simulink model "MPC_Lateral_Control_Model"  (R2021a)
settings: Solver=VariableStepAuto  StartTime=0.0  StopTime=Ts  RelTol=1e-3
InitFcn:
  | MPC_init
StopFcn:
  | simulation_plots_week6
values from neighbouring files (symbols this model uses):
  Vx = 25    [LCA_init.m]    (also in MPC_init.m = 10; week6_init.m = 30)
libraries: mpclib x1
settings Model: Creator=User  LastModifiedBy=User

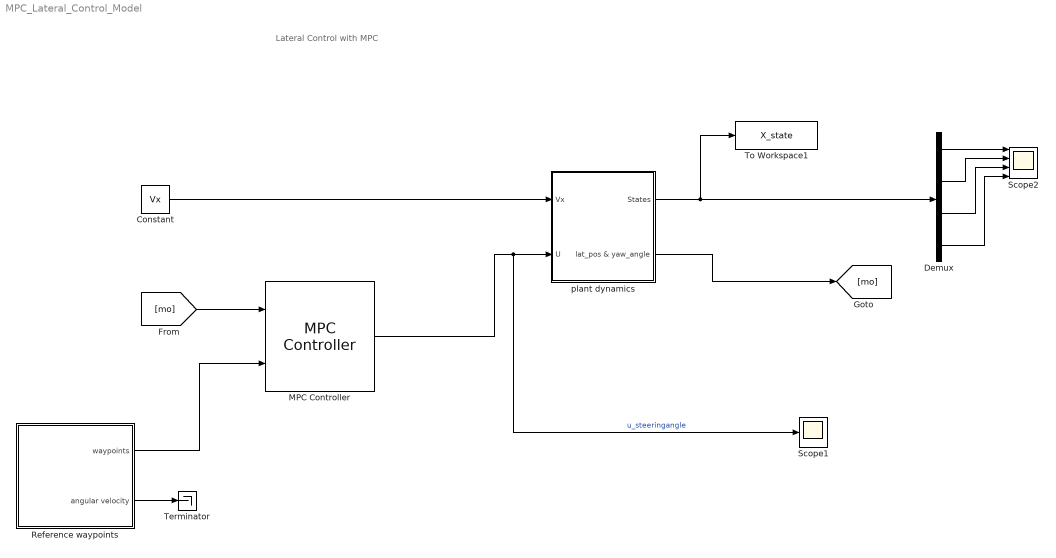
== system MPC_Lateral_Control_Model ==
  note: Lateral Control with MPC
  Constant : Constant  Value=Vx
  Demux : Demux
  MPC Controller : mpclib/MPC Controller  SCDEnableBlockLinearizationSpecification=on  mpcobj=mpc1  is_multiple=0  enable_value=0  return_u0=off  updateMPCinCallerWorkspace=on  md_inport=off  mv_inport=off  uref_inport=off  return_cost=off  return_mvseq=off  return_qpstatus=off  return_xseq=off  return_state=off  return_ovseq=off  state_inport=off  umin_inport=off  umax_inport=off  ymin_inport=off  ymax_inport=off  cc_inport=off  ywt_inport=off  uwt_inport=off  duwt_inport=off  rhoeps_inport=off  pm_inport=off  MaximumP=10  HorizonChoice=FixedHorizon  n_ts=0.1  n_p=10  n_mv=1  n_md=0  n_ud=0  n_mo=2  n_uo=0  BlockDataType=double  SampleTimeInherited=off  switch_inport=off
  Reference waypoints : Subsystem
  Scope1 : Scope
  Scope2 : Scope  NumInputPorts=4
  Terminator : Terminator
  To Workspace1 : ToWorkspace  VariableName=X_state  SampleTime=-1
  plant dynamics : Subsystem
  wires:
  Reference waypoints/1(waypoints) -> MPC Controller/2
  plant dynamics/2(lat_pos & yaw_angle) -> [mo]
  [mo] -> MPC Controller/1
  Constant/1 -> plant dynamics/1(Vx)
  MPC Controller/1 -> Scope1/1, plant dynamics/2(U)  "u_steeringangle"
  plant dynamics/1(States) -> Demux/1, To Workspace1/1
  Reference waypoints/2(angular velocity) -> Terminator/1
  Demux/2 -> Scope2/2
  Demux/3 -> Scope2/3
  Demux/1 -> Scope2/1
  Demux/4 -> Scope2/4

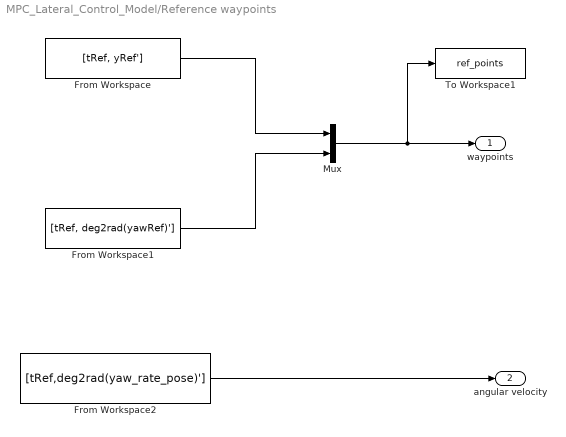
== system MPC_Lateral_Control_Model/Reference waypoints ==
  From Workspace : FromWorkspace  VariableName=[tRef, yRef']  SampleTime=0.1
  From Workspace1 : FromWorkspace  VariableName=[tRef, deg2rad(yawRef)']  SampleTime=0.1
  From Workspace2 : FromWorkspace  VariableName=[tRef,deg2rad(yaw_rate_pose)']  SampleTime=0.1
  Mux : Mux  Inputs=2
  To Workspace1 : ToWorkspace  VariableName=ref_points  SampleTime=-1
  waypoints : Outport
  angular velocity : Outport  Port=2
  wires:
  From Workspace/1 -> Mux/1
  From Workspace1/1 -> Mux/2
  From Workspace2/1 -> angular velocity/1
  Mux/1 -> To Workspace1/1, waypoints/1

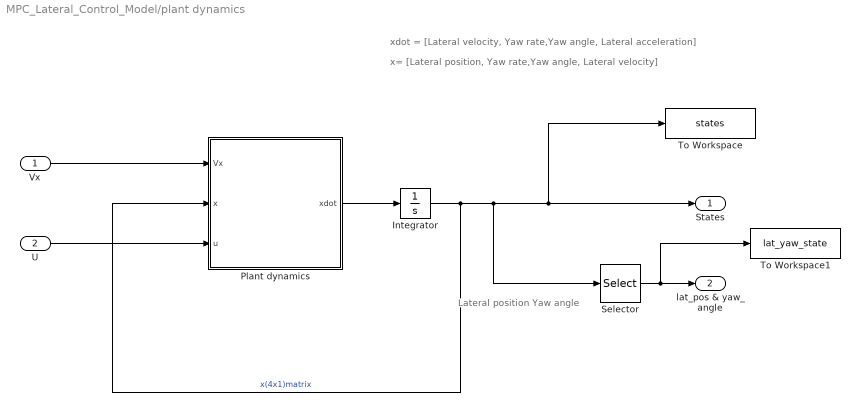
== system MPC_Lateral_Control_Model/plant dynamics ==
  note: Lateral position Yaw angle
  note: x= [Lateral position, Yaw rate,Yaw angle, Lateral velocity]
  note: xdot = [Lateral velocity, Yaw rate,Yaw angle, Lateral acceleration]
  Vx : Inport
  U : Inport  Port=2
  Integrator : Integrator
  Plant dynamics : MATLAB Function  TreatAsAtomicUnit=on
  Selector : Selector  InputPortWidth=4  IndexOptions=Index vector (dialog)  Indices=[1 3]  OutputSizes=1
  To Workspace : ToWorkspace  VariableName=states  SampleTime=-1
  To Workspace1 : ToWorkspace  VariableName=lat_yaw_state  SampleTime=-1
  States : Outport
  lat_pos & yaw_angle : Outport  Port=2
  wires:
  U/1 -> Plant dynamics/3(u)
  Vx/1 -> Plant dynamics/1(Vx)
  Plant dynamics/1(xdot) -> Integrator/1
  Integrator/1 -> Plant dynamics/2(x), Selector/1, To Workspace/1, States/1  "x(4x1)matrix"
  Selector/1 -> To Workspace1/1, lat_pos & yaw_angle/1

== matlab function MPC_Lateral_Control_Model/plant dynamics/Plant dynamics ==
  data: Vx input; x input; u input; xdot output
function xdot = fcn(Vx,x,u)

%% Model parameters
m = 1140;
I_z = 1436.24;%kgm2
l_f = 1.165;
l_r = 1.165;
c_f = 155494.663;% cf for front tire
c_r = 155494.663;% cr for front tire

% assume constant velocity
v_x = Vx;

%% Adding dynamic bicycle model A B C D 
A = [0 1 Vx 0;
    0 -2*(c_f+c_r)/(m*v_x) 0 -2*(l_f*c_f+l_r*c_r)/(m*v_x) - v_x;
    0 0 0 1;
    0 2*(l_r*c_r-l_f*c_f)/(I_z*v_x) 0 -2*(l_r^2*c_r-l_f^2*c_f)/(I_z*v_x)];

B = [0;
    2*c_f/m;
    0;
    2*l_f*c_f/I_z];

C = [1 0 0 0;
    0 1 0 0];

D = [0];

xdot = A*x +B*u;
% y = C*x + D*u;
end
